simulink model "test"  (R2021a)
settings: Solver=VariableStepAuto  StartTime=0.0  StopTime=5  RelTol=1e-3
libraries: simulink x1
settings Model: Creator=majlo  LastModifiedBy=majlo

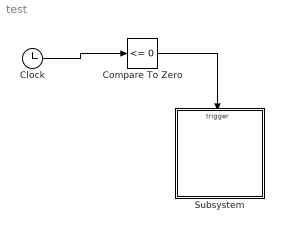
== system test ==
  Clock : Clock
  Compare To Zero : simulink/Logic and Bit Operations/Compare To Zero  relop=<=  OutDataTypeStr=boolean
  Subsystem : Subsystem
  wires:
  Clock/1 -> Compare To Zero/1
  Compare To Zero/1 -> Subsystem/Trigger

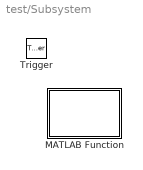
== system test/Subsystem ==
  Trigger : TriggerPort  TriggerType=falling  VariantControl=(inherit)  PortDimensions=1
  MATLAB Function : MATLAB Function  TreatAsAtomicUnit=on

== matlab function test/Subsystem/MATLAB Function ==
function fnc()
    disp("test2");
end
